simulink library "pmm"  (R2021b)
settings: Solver=VariableStepAuto  StartTime=0.0  StopTime=10.0  RelTol=1e-3
undefined symbols (not defined in the file or in its folder): ENUM_ACMAINRLYSTS_OPEN, ENUM_ACPRECHRGRLYSTS_OPEN, ENUM_B2VRLYSTA_OPEN, ENUM_BMSHVSTS_HVOPEN, ENUM_BRAKEPEDAL_RELEASED, ENUM_CACRLYDEM_CLOSE, ENUM_CACRLYSTS_OPEN, ENUM_CHRGFAULT_ACRLYFAIL, ENUM_CHRGFAULT_BCUHVFAIL, ENUM_CHRGFAULT_BCUNEGFAIL, ENUM_CHRGFAULT_BCUTIMEOUT, ENUM_CHRGFAULT_DCDCENABLE, ENUM_CHRGFAULT_DCDCRLYFAIL, ENUM_CHRGFAULT_HVILFAIL, ENUM_CHRGFAULT_PDUHVFAIL, ENUM_CHRGFAULT_RLYCHKFAIL, ENUM_DCDCEACPCURLYSTA_CLOSED, ENUM_DCDCEACPCURLYSTA_FAILTOCLOSE, ENUM_DCDCEACPCURLYSTA_OPEN, ENUM_DCDCEACPCURLYSTA_WELDED, ENUM_DCDCENABLESTS_READY, ENUM_DCDCRLYSTS_OPEN, ENUM_EHPSRLYDEM_CLOSE, ENUM_EHPSRLYSTS_OPEN, ENUM_FOGRLYENCMD_DISABLE, ENUM_GEARACTUALPOSN_D, ENUM_HVPWROFFREQ_POWEROFF, ENUM_KEYSTATUS_OFF, ENUM_KEYSTATUS_ON, ENUM_KEYSTATUS_START, ENUM_LOWBATTVOLTAGE_NORMAL, ENUM_LOWBATTVOLTAGE_POWERDOWN, ENUM_LOWBATTVOLTAGE_POWERUP, ENUM_MCUHVLOOP_POWEROFF, ENUM_MCUHVLOOPSTS_OPEN, ENUM_MCUMAINRLYSTS_OPEN, ENUM_MCUPRECHRGRLYSTS_OPEN, ENUM_PDFAULT_ACRLYOPEN, ENUM_PDFAULT_BCUDISABLE, ENUM_PDFAULT_DCDCDISABLE, ENUM_PDFAULT_DCDCRLYOPEN, ENUM_PDFAULT_EACDISABLE, ENUM_PDFAULT_EACRLYOPEN, ENUM_PDFAULT_EHPSDISABLE, ENUM_PDFAULT_EHPSRLYOPEN, ENUM_PDFAULT_MCUDISABLE, ENUM_PDFAULT_MCUDISCHRG, ENUM_PDFAULT_MCURLYOPEN, ENUM_PEUSELFCHKSTS_NOFAULT, ENUM_PLUGINSTS_NOPLUGIN, ENUM_PLUGINSTS_PLUGIN, ENUM_PMMMODE_DRIVE, ENUM_PMMMODE_LVBATCHRG, ENUM_PUSTATE_DCDCENABLE, ENUM_PUSTATE_EACPRESCHECK, ENUM_PUSTATE_EHPSENABLE, ENUM_PUSTATE_MCUENABLE, ENUM_PUSTATE_PDUMCURLYCLOSED, ENUM_PUSTATE_POWERUPFAIL, ENUM_TARGETGEAR_REVERSE ... (+126)
libraries: hcu_lib x45, simulink x5, ddm x1, dsc x1
(part 7 of 7)

== stateflow chart pmm/PMM/PowerModeManagement/PMM Switch Enum Creator/ChrgFault_SW/cycle time setting ==
  state cycle_time_setting
    en:
    counter = 0;
    (default) -> (junction 182) : {
        | trig;
        | counter++;
        | }
    cycle_time_setting -> (junction 182) : {counter++;}
    (junction 182) -> (junction 6)
    (junction 6) -> (junction 38) [order 1] : [counter >= trig_cnt]
    (junction 6) -> (junction 44) [order 2]
    (junction 38) -> (junction 40) : {
        | trig;
        | counter = 0;
        | }
    (junction 40) -> (junction 44)
    (junction 44) -> (junction 211)
  data: counter local uint32; trig_cnt input
  events: trig output FUNCTION_CALL_EVENT

== stateflow chart pmm/PMM/PowerModeManagement/PMM Switch Enum Creator/PowerDownFault_SW/Subsystem/Chart ==
  state sw
    en:
    a_flg = FALSE ;
    b_flg = FALSE;
    c_flg = FALSE;
    d_flg = FALSE;
    e_flg = FALSE;
    f_flg = FALSE;
    g_flg = FALSE;
    h_flg = FALSE;
    i_flg = FALSE;
    j_flg = FALSE;
    k_flg = FALSE;
    du:
    cnt = a_in+b_in+c_in+d_in+e_in+f_in+g_in+h_in+i_in+j_in+k_in;
    (default) -> (junction 138)
    sw -> (junction 138)
    (junction 138) -> (junction 141) [order 1] : [a_in && !a_flg]
    (junction 138) -> (junction 134) [order 2]
    (junction 141) -> (junction 137) : {OUT_enum = a_enum;
        | a_flg =TRUE;
        | cnt1 = cnt1 + 1;}
    (junction 134) -> (junction 132) [order 1] : [b_in && !b_flg]
    (junction 134) -> (junction 139) [order 2]
    (junction 132) -> (junction 127) : {OUT_enum = b_enum;
        | b_flg =TRUE;
        | cnt1 = cnt1 + 1;}
    (junction 139) -> (junction 140) [order 1] : [c_in && !c_flg]
    (junction 139) -> (junction 143) [order 2]
    (junction 140) -> (junction 142) : {OUT_enum = c_enum;
        | c_flg =TRUE;
        | cnt1 = cnt1 + 1;}
    (junction 143) -> (junction 144) [order 1] : [d_in && !d_flg]
    (junction 143) -> (junction 135) [order 2]
    (junction 144) -> (junction 133) : {OUT_enum = d_enum;
        | d_flg =TRUE;
        | cnt1 = cnt1 + 1;}
    (junction 135) -> (junction 136) [order 1] : [e_in && !e_flg]
    (junction 135) -> (junction 124) [order 2]
    (junction 136) -> (junction 123) : {OUT_enum = e_enum;
        | e_flg =TRUE;
        | cnt1 = cnt1 + 1;}
    (junction 124) -> (junction 125) [order 1] : [f_in && !f_flg]
    (junction 124) -> (junction 128) [order 2]
    (junction 125) -> (junction 126) : {OUT_enum = f_enum;
        | f_flg =TRUE;
        | cnt1 = cnt1 + 1;}
    (junction 128) -> (junction 129) [order 1] : [g_in && !g_flg]
    (junction 128) -> (junction 131) [order 2]
    (junction 129) -> (junction 130) : {OUT_enum = g_enum;
        | g_flg =TRUE;
        | cnt1 = cnt1 + 1;}
    (junction 131) -> (junction 159) [order 1] : [h_in && !h_flg]
    (junction 131) -> (junction 147) [order 2]
    (junction 159) -> (junction 149) : {OUT_enum = h_enum;
        | h_flg =TRUE;
        | cnt1 = cnt1 + 1;}
    (junction 147) -> (junction 162) [order 1] : [i_in && !i_flg]
    (junction 147) -> (junction 148) [order 2]
    (junction 162) -> (junction 155) : {OUT_enum = i_enum;
        | i_flg =TRUE;
        | cnt1 = cnt1 + 1;}
    (junction 148) -> (junction 161) [order 1] : [j_in && !j_flg]
    (junction 148) -> (junction 150) [order 2]
    (junction 161) -> (junction 163) : {OUT_enum = j_enum;
        | j_flg =TRUE;
        | cnt1 = cnt1 + 1;}
    (junction 150) -> (junction 166) [order 1] : [k_in && !k_flg]
    (junction 150) -> (junction 195) [order 2]
    (junction 166) -> (junction 151) : {OUT_enum = k_enum;
        | k_flg =TRUE;
        | cnt1 = cnt1 + 1;}
    (junction 195) -> (junction 202) [order 2] : [cnt == cnt1]
    (junction 195) -> (junction 196) [order 1] : [cnt == 0]
    (junction 202) -> (junction 203) : {
        | a_flg = FALSE ;
        | b_flg = FALSE;
        | c_flg = FALSE;
        | d_flg = FALSE;
        | e_flg = FALSE;
        | f_flg = FALSE;
        | g_flg = FALSE;
        | h_flg = FALSE;
        | i_flg = FALSE;
        | j_flg = FALSE;
        | k_flg = FALSE;
        | cnt1 = 0;
        | }
    (junction 195) -> (junction 193) [order 3] : {cnt1 = cnt;}
    (junction 196) -> (junction 194) : {OUT_enum = 0}
  (default) -> sw
  data: a_in input boolean; b_in input boolean; c_in input boolean; OUT_enum output uint8; a_flg local boolean; b_flg local boolean; c_flg local boolean; d_in input boolean; d_flg local boolean; e_in input; f_in input; g_in input; h_in input; i_in input; j_in input; k_in input; a_enum input; b_enum input; c_enum input; d_enum input; e_enum input; e_flg local boolean size=1; cnt local uint32 size=1; f_enum input; g_enum input; h_enum input; i_enum input; j_enum input; k_enum input; f_flg local boolean size=1; g_flg local boolean size=1; h_flg local boolean size=1; i_flg local boolean size=1; j_flg local boolean size=1; k_flg local boolean size=1; cnt1 local uint32; FALSE parameter; TRUE parameter

== stateflow chart pmm/PMM/PowerModeManagement/PMM Flag Creator /Low Battery Voltage/Low Voltage Charge Action Flasher/Brake Lamp  Flasher/Chart ==
  state init
    en:
    time_cnt = 0;
    ON_flg = TRUE;
    OFF_flg = FALSE;
    out = 0;
    CycleCnt_cnt = 0;
  state OFF
    en:
    out = 0;
    time_cnt = 0;
    OFF -> (junction 38) [order 1]
    (junction 38) -> OFF : {time_cnt = time_cnt + 1;}
  state ON
    en:
    out = 1;
    time_cnt = 0;
    du:
    time_cnt = time_cnt +1;
  state WAIT
    en:
    out = 0;
    time_cnt = 0;
    du:
    time_cnt = time_cnt + 1;
  (default) -> init
  init -> (junction 57)
  (junction 57) -> ON : [ON_flg]
  OFF -> (junction 46) [order 2] : [time_cnt > OFF_cnt]
  (junction 46) -> (junction 47) : {time_cnt = 0; ON_flg = TRUE; OFF_flg = FALSE; CycleCnt_cnt = CycleCnt_cnt +1;}
  (junction 47) -> ON : [ON_flg]
  ON -> (junction 44) : [time_cnt > ON_cnt]
  (junction 44) -> (junction 42) : {time_cnt = 0; ON_flg = FALSE; OFF_flg = TRUE;}
  (junction 42) -> OFF : [OFF_flg]
  OFF -> (junction 66) [order 1] : [time_cnt > OFF_cnt && CycleCnt_cnt >= Cycle_cnt]
  (junction 66) -> WAIT : {time_cnt = 0;}
  (junction 62) -> ON : {time_cnt = 0; ON_flg = TRUE; OFF_flg = FALSE; CycleCnt_cnt = 0;}
  WAIT -> (junction 62) : [time_cnt >= WAIT_cnt]
  data: ON_cnt input uint32; OFF_cnt input uint32; WAIT_cnt input uint32; Cycle_cnt input uint32; out output uint8; time_cnt local uint32; OFF_flg local boolean; ON_flg local boolean; CycleCnt_cnt local uint32; FALSE parameter; TRUE parameter

== stateflow chart pmm/PMM/PowerModeManagement/PMM Flag Creator /Low Battery Voltage/Low Voltage Charge Action Flasher/Reverse Buzzer Flasher/Chart ==
  state init
    en:
    time_cnt = 0;
    ON_flg = TRUE;
    OFF_flg = FALSE;
    out = 0;
    CycleCnt_cnt = 0;
  state OFF
    en:
    out = 0;
    time_cnt = 0;
    OFF -> (junction 38) [order 1]
    (junction 38) -> OFF : {time_cnt = time_cnt + 1;}
  state ON
    en:
    out = 1;
    time_cnt = 0;
    du:
    time_cnt = time_cnt +1;
  state WAIT
    en:
    out = 0;
    time_cnt = 0;
    du:
    time_cnt = time_cnt + 1;
  (default) -> init
  init -> (junction 57)
  (junction 57) -> ON : [ON_flg]
  OFF -> (junction 46) [order 2] : [time_cnt > OFF_cnt]
  (junction 46) -> (junction 47) : {time_cnt = 0; ON_flg = TRUE; OFF_flg = FALSE; CycleCnt_cnt = CycleCnt_cnt +1;}
  (junction 47) -> ON : [ON_flg]
  ON -> (junction 44) : [time_cnt > ON_cnt]
  (junction 44) -> (junction 42) : {time_cnt = 0; ON_flg = FALSE; OFF_flg = TRUE;}
  (junction 42) -> OFF : [OFF_flg]
  OFF -> (junction 66) [order 1] : [time_cnt > OFF_cnt && CycleCnt_cnt >= Cycle_cnt]
  (junction 66) -> WAIT : {time_cnt = 0;}
  (junction 62) -> ON : {time_cnt = 0; ON_flg = TRUE; OFF_flg = FALSE; CycleCnt_cnt = 0;}
  WAIT -> (junction 62) : [time_cnt >= WAIT_cnt]
  data: ON_cnt input uint32; OFF_cnt input uint32; WAIT_cnt input uint32; Cycle_cnt input uint32; out output uint8; time_cnt local uint32; OFF_flg local boolean; ON_flg local boolean; CycleCnt_cnt local uint32; FALSE parameter; TRUE parameter

== stateflow chart pmm/PMM/PowerModeManagement/PMM Switch Enum Creator/PowerDownFault_SW/cycle time setting ==
  state cycle_time_setting
    en:
    counter = 0;
    (default) -> (junction 182) : {
        | trig;
        | counter++;
        | }
    cycle_time_setting -> (junction 182) : {counter++;}
    (junction 182) -> (junction 6)
    (junction 6) -> (junction 38) [order 1] : [counter >= trig_cnt]
    (junction 6) -> (junction 44) [order 2]
    (junction 38) -> (junction 40) : {
        | trig;
        | counter = 0;
        | }
    (junction 40) -> (junction 44)
    (junction 44) -> (junction 211)
  data: counter local uint32; trig_cnt input
  events: trig output FUNCTION_CALL_EVENT

== stateflow chart pmm/PMM/PowerModeManagement/PMM Switch Enum Creator/PowerUpState_SW/PowerUpState_SW ==
  state sw1
    en:
    a_flg = FALSE ;
    b_flg = FALSE;
    c_flg = FALSE;
    d_flg = FALSE;
    e_flg = FALSE;
    du:
    cnt = a_in+b_in+c_in+d_in+e_in;
    (default) -> (junction 110)
    sw1 -> (junction 110)
    (junction 110) -> (junction 124) [order 1] : [a_in && !a_flg]
    (junction 110) -> (junction 116) [order 2]
    (junction 124) -> (junction 109) : {OUT_enum = a_enum;
        | a_flg =TRUE;
        | cnt1 = cnt1 + 1;}
    (junction 116) -> (junction 114) [order 1] : [b_in && !b_flg]
    (junction 116) -> (junction 123) [order 2]
    (junction 114) -> (junction 107) : {OUT_enum = b_enum;
        | b_flg =TRUE;
        | cnt1 = cnt1 + 1;}
    (junction 123) -> (junction 125) [order 1] : [c_in && !c_flg]
    (junction 123) -> (junction 131) [order 2]
    (junction 125) -> (junction 122) : {OUT_enum = c_enum;
        | c_flg =TRUE;
        | cnt1 = cnt1 + 1;}
    (junction 131) -> (junction 120) [order 1] : [d_in && !d_flg]
    (junction 131) -> (junction 115) [order 2]
    (junction 120) -> (junction 108) : {OUT_enum = d_enum;
        | d_flg =TRUE;
        | cnt1 = cnt1 + 1;}
    (junction 115) -> (junction 117) [order 1] : [e_in && !e_flg]
    (junction 115) -> (junction 80) [order 2]
    (junction 117) -> (junction 103) : {OUT_enum = e_enum;
        | e_flg =TRUE;
        | cnt1 = cnt1 + 1;}
    (junction 80) -> (junction 139) [order 2] : [cnt == cnt1]
    (junction 80) -> (junction 79) [order 1] : [cnt == 0]
    (junction 139) -> (junction 141) : {
        | a_flg = FALSE ;
        | b_flg = FALSE;
        | c_flg = FALSE;
        | d_flg = FALSE;
        | e_flg = FALSE;;
        | cnt1 = 0;
        | }
    (junction 80) -> (junction 156) [order 3] : {cnt1 = cnt;}
    (junction 79) -> (junction 135) : {OUT_enum = Sys_in}
  (default) -> sw1
  data: Sys_in input uint8 size=1; a_in input boolean size=1; b_in input boolean size=1; c_in input boolean size=1; OUT_enum output uint8 size=1; a_flg local boolean size=1; b_flg local boolean size=1; c_flg local boolean size=1; d_in input boolean size=1; d_flg local boolean size=1; e_in input boolean size=1; a_enum input uint8 size=1; b_enum input uint8 size=1; c_enum input uint8 size=1; d_enum input uint8 size=1; e_enum input uint8 size=1; e_flg local boolean size=1; cnt local uint32 size=1; cnt1 local uint32; FALSE parameter; TRUE parameter

== stateflow chart pmm/PMM/PowerModeManagement/PMM Switch Enum Creator/cycle time setting ==
  state cycle_time_setting
    en:
    counter = 0;
    (default) -> (junction 182) : {
        | trig;
        | counter++;
        | }
    cycle_time_setting -> (junction 182) : {counter++;}
    (junction 182) -> (junction 6)
    (junction 6) -> (junction 38) [order 1] : [counter >= trig_cnt]
    (junction 6) -> (junction 44) [order 2]
    (junction 38) -> (junction 40) : {
        | trig;
        | counter = 0;
        | }
    (junction 40) -> (junction 44)
    (junction 44) -> (junction 211)
  data: counter local uint32; trig_cnt input
  events: trig output FUNCTION_CALL_EVENT

== stateflow chart pmm/PMM/PowerModeManagement/PMM Flag Creator /Low Battery Voltage/Long Idle Flasher/Reverse Buzzer Flasher/Chart ==
  state init
    en:
    time_cnt = 0;
    ON_flg = TRUE;
    OFF_flg = FALSE;
    out = 0;
    CycleCnt_cnt = 0;
  state OFF
    en:
    out = 0;
    time_cnt = 0;
    OFF -> (junction 38) [order 1]
    (junction 38) -> OFF : {time_cnt = time_cnt + 1;}
  state ON
    en:
    out = 1;
    time_cnt = 0;
    du:
    time_cnt = time_cnt +1;
  state WAIT
    en:
    out = 0;
    time_cnt = 0;
    du:
    time_cnt = time_cnt + 1;
  (default) -> init
  init -> (junction 57)
  (junction 57) -> ON : [ON_flg]
  OFF -> (junction 46) [order 2] : [time_cnt > OFF_cnt]
  (junction 46) -> (junction 47) : {time_cnt = 0; ON_flg = TRUE; OFF_flg = FALSE; CycleCnt_cnt = CycleCnt_cnt +1;}
  (junction 47) -> ON : [ON_flg]
  ON -> (junction 44) : [time_cnt > ON_cnt]
  (junction 44) -> (junction 42) : {time_cnt = 0; ON_flg = FALSE; OFF_flg = TRUE;}
  (junction 42) -> OFF : [OFF_flg]
  OFF -> (junction 66) [order 1] : [time_cnt > OFF_cnt && CycleCnt_cnt >= Cycle_cnt]
  (junction 66) -> WAIT : {time_cnt = 0;}
  (junction 62) -> ON : {time_cnt = 0; ON_flg = TRUE; OFF_flg = FALSE; CycleCnt_cnt = 0;}
  WAIT -> (junction 62) : [time_cnt >= WAIT_cnt]
  data: ON_cnt input uint32; OFF_cnt input uint32; WAIT_cnt input uint32; Cycle_cnt input uint32; out output uint8; time_cnt local uint32; OFF_flg local boolean; ON_flg local boolean; CycleCnt_cnt local uint32; FALSE parameter; TRUE parameter

== stateflow chart pmm/PMM/PowerModeManagement/PMM_SCP/LifeCounter ==
  state counter_calculation
    (default) -> (junction 54) : {
        | counter = 0;
        | VPMM_VCULife1_cnt = 0;
        | VPMM_VCULife2_cnt = 0;
        | VPMM_V2BLifeSig_cnt = 0;
        | }
    counter_calculation -> (junction 54) : {
        | counter++;
        | VPMM_VCULife1_cnt++;
        | }
    (junction 54) -> (junction 55) [order 1] : [(counter %%10) ==0 /*100ms*/]
    (junction 55) -> (junction 56) : {
        | VPMM_VCULife2_cnt++;
        | VPMM_V2BLifeSig_cnt++;
        | }
    (junction 54) -> (junction 57) [order 2]
    (junction 56) -> (junction 57)
    (junction 57) -> (junction 4)
    (junction 4) -> (junction 9) [order 1] : [VPMM_VCULife1_cnt > 255]
    (junction 4) -> (junction 13) [order 2]
    (junction 9) -> (junction 11) : {
        | VPMM_VCULife1_cnt = 0;
        | }
    (junction 11) -> (junction 13)
    (junction 13) -> (junction 16)
    (junction 16) -> (junction 18) [order 1] : [VPMM_VCULife2_cnt > 255]
    (junction 18) -> (junction 20) : {
        | VPMM_VCULife2_cnt = 0;
        | }
    (junction 16) -> (junction 22) [order 2]
    (junction 20) -> (junction 22)
    (junction 22) -> (junction 25)
    (junction 25) -> (junction 27) [order 1] : [VPMM_V2BLifeSig_cnt > 255]
    (junction 27) -> (junction 30) : {
        | VPMM_V2BLifeSig_cnt = 0;
        | counter = 0;
        | }
    (junction 25) -> (junction 31) [order 2]
    (junction 30) -> (junction 31)
    (junction 31) -> (junction 42)
  data: VPMM_VCULife1_cnt output double; VPMM_VCULife2_cnt output double; counter local double; VPMM_V2BLifeSig_cnt output double
